simulink model "TranslationalDynamics"  (R2018b)
settings: Solver=FixedStepAuto  StartTime=0.0  StopTime=50  FixedStep=0.005  RelTol=1e-3
InitFcn:
  | loadThrusterData
undefined symbols (not defined in the file or in its folder): DiscIntNeverNeededParam
settings Model: Creator=Andy  LastModifiedBy=Andy
settings DataIOCC: SaveOutput=off  SaveTime=off
settings ModelReferenceCC: ModelReferenceNumInstancesAllowed=Single
settings RTWCC: GenCodeOnly=on

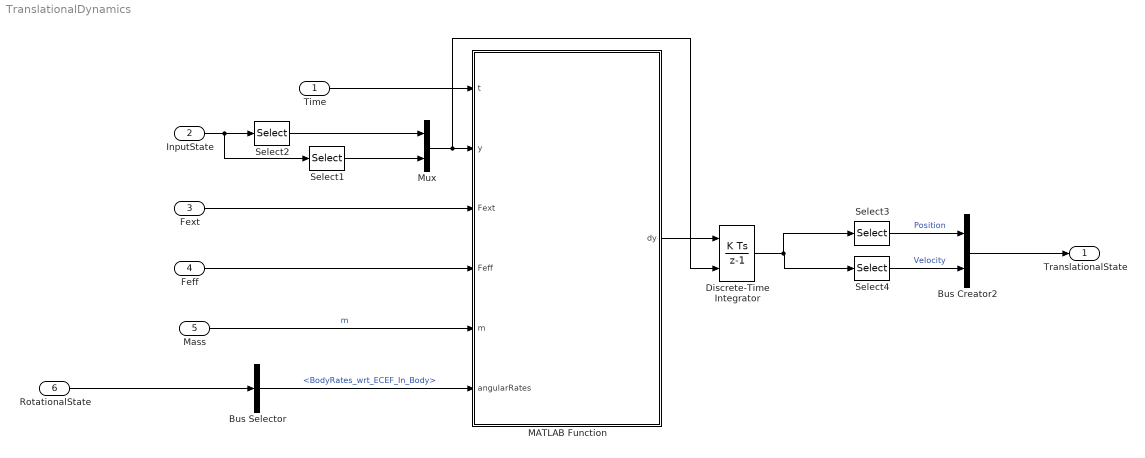
== system TranslationalDynamics ==
  Time : Inport  OutDataTypeStr=double  PortDimensions=1
  InputState : Inport  Port=2  OutDataTypeStr=double
  Fext : Inport  Port=3  OutDataTypeStr=double  PortDimensions=3
  Feff : Inport  Port=4  OutDataTypeStr=double  PortDimensions=3
  Mass : Inport  Port=5  OutDataTypeStr=double  PortDimensions=1
  RotationalState : Inport  Port=6  OutDataTypeStr=Bus: RotStateBodyECEFBus
  Bus Creator2 : BusCreator  Inputs=2  OutDataTypeStr=Bus: TranStateBodyBus
      settings: InheritFromInputs=off
  Bus Selector : BusSelector  OutputSignals=BodyRates_wrt_ECEF_In_Body
  Discrete-Time Integrator : DiscreteIntegrator  InitialConditionSource=external  SampleTime=-1  ICPrevOutput=DiscIntNeverNeededParam  ICPrevScaledInput=DiscIntNeverNeededParam
  MATLAB Function : MATLAB Function  TreatAsAtomicUnit=on
  Mux : Mux  Inputs=2
  Select1 : Selector  InputPortWidth=6  IndexOptions=Index vector (dialog)  Indices=[4:6]  OutputSizes=1
  Select2 : Selector  InputPortWidth=6  IndexOptions=Index vector (dialog)  Indices=[1:3]  OutputSizes=1
  Select3 : Selector  InputPortWidth=6  IndexOptions=Index vector (dialog)  Indices=[1:3]  OutputSizes=1
  Select4 : Selector  InputPortWidth=6  IndexOptions=Index vector (dialog)  Indices=[4:6]  OutputSizes=1
  TranslationalState : Outport  OutDataTypeStr=Bus: TranStateBodyBus
  wires:
  MATLAB Function/1(dy) -> Discrete-Time Integrator/1
  Discrete-Time Integrator/1 -> Select3/1, Select4/1
  Time/1 -> MATLAB Function/1(t)
  Mass/1 -> MATLAB Function/5(m)  "m"
  Mux/1 -> Discrete-Time Integrator/2, MATLAB Function/2(y)
  Select2/1 -> Mux/1
  Select1/1 -> Mux/2
  RotationalState/1 -> Bus Selector/1
  Feff/1 -> MATLAB Function/4(Feff)
  Fext/1 -> MATLAB Function/3(Fext)
  InputState/1 -> Select1/1, Select2/1
  Bus Creator2/1 -> TranslationalState/1
  Select3/1 -> Bus Creator2/1  "Position"
  Select4/1 -> Bus Creator2/2  "Velocity"
  Bus Selector/1 -> MATLAB Function/6(angularRates)  "<BodyRates_wrt_ECEF_In_Body>"

== matlab function TranslationalDynamics/MATLAB Function ==
  data: t input; dy output; y input; Fext input; Feff input; m input; angularRates input
function dy = calltranslationalEOM(t,y,Fext,Feff,m,angularRates)

 dy = translationalEOM(t,y,Fext,Feff,m,angularRates);
